simulink model "stage_1"  (Simulink 8.7)
settings: Solver=VariableStepAuto  StartTime=0.0  StopTime=.01  FixedStep=.000295  MaxStep=.000059  RelTol=1e-3
settings Model: Creator=eispin  LastModifiedBy=eispin  PauseTimes=0
settings DataIOCC: LimitDataPoints=off  SaveFormat=Dataset
settings DebuggingCC: UnderspecifiedInitializationDetection=Simplified  MergeDetectMultiDrivingBlocksExec=error
settings HardwareCC: ProdBitPerPointer=64  ProdLargestAtomicFloat=Float  ProdIntDivRoundTo=Zero  ProdEndianess=LittleEndian  ProdWordSize=64  ProdHWDeviceType=Intel->x86-64 (Windows64)
settings ModelReferenceCC: PropagateSignalLabelsOutOfModel=on
settings ConfigComp: CovModelRefEnable=off

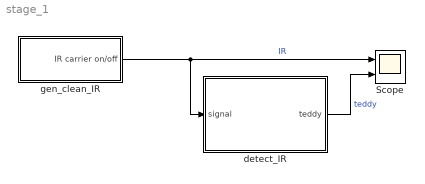
== system stage_1 ==
  Scope : Scope  NumInputPorts=2
  detect_IR : Stateflow chart  TreatAsAtomicUnit=on
  gen_clean_IR : Subsystem
  wires:
  gen_clean_IR/1(IR carrier on/off) -> detect_IR/1(signal), Scope/1  "IR"
  detect_IR/1(teddy) -> Scope/2  "teddy"

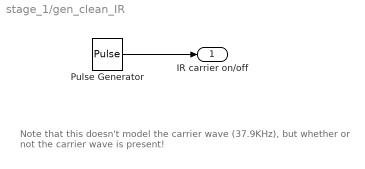
== system stage_1/gen_clean_IR ==
  note: Note that this doesn't model the carrier wave (37.9KHz),
      | but whether or not the carrier wave is present!
  Pulse Generator : DiscretePulseGenerator  PulseType=Time based  Period=.001180  PulseWidth=50
  IR carrier on/off : Outport
  wires:
  Pulse Generator/1 -> IR carrier on/off/1

== stateflow chart detect_IR ==
  state NoTeddy
    % signal is 1,
    % waiting for 0
    entry:
    teddy = 0
  state Something
    % signal is 0,
    % waiting for 1
    entry:
    % don't change teddy
  note: Note that the "signal" must be treated as inverted,
      | so '0' is "carrier detected" and '1' is "carrier absent"
  state WasTeddy
    % signal is 1
    % waiting for 0
    entry:
    teddy = 1
  state TooMuch
    % signal is 0,
    % waiting for 1
    entry:
    teddy = 0
  state ConfirmZero
  state ConfirmOne
  (default) -> NoTeddy
  ConfirmZero -> Something [order 1] : [after(590-tolerance, usec)]
  NoTeddy -> ConfirmZero : [signal < .5]
  ConfirmZero -> NoTeddy [order 2] : [signal > .5]
  WasTeddy -> ConfirmZero [order 2] : [signal < .5]
  Something -> ConfirmOne [order 2] : [signal > .5]
  Something -> TooMuch [order 1] : [after(2*tolerance, usec)]
  TooMuch -> NoTeddy : [signal > .5]
  WasTeddy -> NoTeddy [order 1] : [after(2*tolerance, usec)]
  ConfirmOne -> TooMuch [order 2] : [signal < .5]
  ConfirmOne -> WasTeddy [order 1] : [after(590-tolerance, usec)]
  data: signal input double; tolerance constant double =60; teddy output double
  data tolerance settings: description=MUST be bigger than the simulation stepsize
